simulink model "gm_parallel_lht"  (R2019b)
settings: Solver=FixedStepDiscrete  StartTime=0.0  StopTime=inf  RelTol=1e-3
undefined symbols (not defined in the file or in its folder): bt, height, width
libraries: hdlsllib x190, simulink x13, hdlmdlgenlib x7, dspsrcs4 x1
(part 8 of 18)

== system gm_parallel_lht/Parallel LHT/Parallel LHT Accumulator/Accumulator with Switches/Accumulator_instance72 ==
  mode : Inport  OutDataTypeStr=boolean  PortDimensions=1  SampleTime=6.66666666666667e-09
  address : Inport  Port=2  OutDataTypeStr=fixdt(0, 11, 0)  PortDimensions=1  SampleTime=6.66666666666667e-09
  edge : Inport  Port=3  OutDataTypeStr=boolean  PortDimensions=1  SampleTime=6.66666666666667e-09
  AND : Logic  IconShape=distinctive  AllPortsSameDT=off  OutDataTypeStr=boolean
  Add : Sum  OutDataTypeStr=fixdt(0, ceil(log2(maxRho*2)), 0)
  Block RAM : Subsystem
  Delay{,1..3} (4 alike) : Delay  DelayLength=1
  Multiport Switch : MultiPortSwitch  DataPortOrder=Zero-based contiguous  Inputs=2  zeroidx=on
  Multiport Switch1 : MultiPortSwitch  DataPortOrder=Zero-based contiguous  Inputs=2  zeroidx=on
  Relational Operator : RelationalOperator  Operator===  OutDataTypeStr=boolean  RndMeth=Simplest
  Vote : Constant  OutDataTypeStr=fixdt(0,1,0)  SampleTime=-1
  Zero : Constant  OutDataTypeStr=fixdt(0,1,0)  SampleTime=-1
  hps : Outport
  wires:
  Add/1 -> Delay3/1, Multiport Switch/3
  Multiport Switch1/1 -> Add/2
  Delay3/1 -> Multiport Switch1/3
  Multiport Switch/1 -> Block RAM/1(wr_data)
  edge/1 -> Delay1/1
  address/1 -> Block RAM/4(rd_addr), Delay/1, Relational Operator/2
  mode/1 -> Multiport Switch/1
  AND/1 -> Delay2/1
  Block RAM/1(rd_data) -> Multiport Switch1/2, hps/1
  Delay/1 -> Block RAM/2(wr_addr), Relational Operator/1
  Delay1/1 -> Block RAM/3(wr_en), AND/1
  Delay2/1 -> Multiport Switch1/1
  Relational Operator/1 -> AND/2
  Vote/1 -> Add/1
  Zero/1 -> Multiport Switch/2

== system gm_parallel_lht/Parallel LHT/Parallel LHT Accumulator/Accumulator with Switches/Accumulator_instance73 ==
  mode : Inport  OutDataTypeStr=boolean  PortDimensions=1  SampleTime=6.66666666666667e-09
  address : Inport  Port=2  OutDataTypeStr=fixdt(0, 11, 0)  PortDimensions=1  SampleTime=6.66666666666667e-09
  edge : Inport  Port=3  OutDataTypeStr=boolean  PortDimensions=1  SampleTime=6.66666666666667e-09
  AND : Logic  IconShape=distinctive  AllPortsSameDT=off  OutDataTypeStr=boolean
  Add : Sum  OutDataTypeStr=fixdt(0, ceil(log2(maxRho*2)), 0)
  Block RAM : Subsystem
  Delay{,1..3} (4 alike) : Delay  DelayLength=1
  Multiport Switch : MultiPortSwitch  DataPortOrder=Zero-based contiguous  Inputs=2  zeroidx=on
  Multiport Switch1 : MultiPortSwitch  DataPortOrder=Zero-based contiguous  Inputs=2  zeroidx=on
  Relational Operator : RelationalOperator  Operator===  OutDataTypeStr=boolean  RndMeth=Simplest
  Vote : Constant  OutDataTypeStr=fixdt(0,1,0)  SampleTime=-1
  Zero : Constant  OutDataTypeStr=fixdt(0,1,0)  SampleTime=-1
  hps : Outport
  wires:
  Add/1 -> Delay3/1, Multiport Switch/3
  Multiport Switch1/1 -> Add/2
  Delay3/1 -> Multiport Switch1/3
  Multiport Switch/1 -> Block RAM/1(wr_data)
  edge/1 -> Delay1/1
  address/1 -> Block RAM/4(rd_addr), Delay/1, Relational Operator/2
  mode/1 -> Multiport Switch/1
  AND/1 -> Delay2/1
  Block RAM/1(rd_data) -> Multiport Switch1/2, hps/1
  Delay/1 -> Block RAM/2(wr_addr), Relational Operator/1
  Delay1/1 -> Block RAM/3(wr_en), AND/1
  Delay2/1 -> Multiport Switch1/1
  Relational Operator/1 -> AND/2
  Vote/1 -> Add/1
  Zero/1 -> Multiport Switch/2

== system gm_parallel_lht/Parallel LHT/Parallel LHT Accumulator/Accumulator with Switches/Accumulator_instance74 ==
  mode : Inport  OutDataTypeStr=boolean  PortDimensions=1  SampleTime=6.66666666666667e-09
  address : Inport  Port=2  OutDataTypeStr=fixdt(0, 11, 0)  PortDimensions=1  SampleTime=6.66666666666667e-09
  edge : Inport  Port=3  OutDataTypeStr=boolean  PortDimensions=1  SampleTime=6.66666666666667e-09
  AND : Logic  IconShape=distinctive  AllPortsSameDT=off  OutDataTypeStr=boolean
  Add : Sum  OutDataTypeStr=fixdt(0, ceil(log2(maxRho*2)), 0)
  Block RAM : Subsystem
  Delay{,1..3} (4 alike) : Delay  DelayLength=1
  Multiport Switch : MultiPortSwitch  DataPortOrder=Zero-based contiguous  Inputs=2  zeroidx=on
  Multiport Switch1 : MultiPortSwitch  DataPortOrder=Zero-based contiguous  Inputs=2  zeroidx=on
  Relational Operator : RelationalOperator  Operator===  OutDataTypeStr=boolean  RndMeth=Simplest
  Vote : Constant  OutDataTypeStr=fixdt(0,1,0)  SampleTime=-1
  Zero : Constant  OutDataTypeStr=fixdt(0,1,0)  SampleTime=-1
  hps : Outport
  wires:
  Add/1 -> Delay3/1, Multiport Switch/3
  Multiport Switch1/1 -> Add/2
  Delay3/1 -> Multiport Switch1/3
  Multiport Switch/1 -> Block RAM/1(wr_data)
  edge/1 -> Delay1/1
  address/1 -> Block RAM/4(rd_addr), Delay/1, Relational Operator/2
  mode/1 -> Multiport Switch/1
  AND/1 -> Delay2/1
  Block RAM/1(rd_data) -> Multiport Switch1/2, hps/1
  Delay/1 -> Block RAM/2(wr_addr), Relational Operator/1
  Delay1/1 -> Block RAM/3(wr_en), AND/1
  Delay2/1 -> Multiport Switch1/1
  Relational Operator/1 -> AND/2
  Vote/1 -> Add/1
  Zero/1 -> Multiport Switch/2

== system gm_parallel_lht/Parallel LHT/Parallel LHT Accumulator/Accumulator with Switches/Accumulator_instance75 ==
  mode : Inport  OutDataTypeStr=boolean  PortDimensions=1  SampleTime=6.66666666666667e-09
  address : Inport  Port=2  OutDataTypeStr=fixdt(0, 11, 0)  PortDimensions=1  SampleTime=6.66666666666667e-09
  edge : Inport  Port=3  OutDataTypeStr=boolean  PortDimensions=1  SampleTime=6.66666666666667e-09
  AND : Logic  IconShape=distinctive  AllPortsSameDT=off  OutDataTypeStr=boolean
  Add : Sum  OutDataTypeStr=fixdt(0, ceil(log2(maxRho*2)), 0)
  Block RAM : Subsystem
  Delay{,1..3} (4 alike) : Delay  DelayLength=1
  Multiport Switch : MultiPortSwitch  DataPortOrder=Zero-based contiguous  Inputs=2  zeroidx=on
  Multiport Switch1 : MultiPortSwitch  DataPortOrder=Zero-based contiguous  Inputs=2  zeroidx=on
  Relational Operator : RelationalOperator  Operator===  OutDataTypeStr=boolean  RndMeth=Simplest
  Vote : Constant  OutDataTypeStr=fixdt(0,1,0)  SampleTime=-1
  Zero : Constant  OutDataTypeStr=fixdt(0,1,0)  SampleTime=-1
  hps : Outport
  wires:
  Add/1 -> Delay3/1, Multiport Switch/3
  Multiport Switch1/1 -> Add/2
  Delay3/1 -> Multiport Switch1/3
  Multiport Switch/1 -> Block RAM/1(wr_data)
  edge/1 -> Delay1/1
  address/1 -> Block RAM/4(rd_addr), Delay/1, Relational Operator/2
  mode/1 -> Multiport Switch/1
  AND/1 -> Delay2/1
  Block RAM/1(rd_data) -> Multiport Switch1/2, hps/1
  Delay/1 -> Block RAM/2(wr_addr), Relational Operator/1
  Delay1/1 -> Block RAM/3(wr_en), AND/1
  Delay2/1 -> Multiport Switch1/1
  Relational Operator/1 -> AND/2
  Vote/1 -> Add/1
  Zero/1 -> Multiport Switch/2

== system gm_parallel_lht/Parallel LHT/Parallel LHT Accumulator/Accumulator with Switches/Accumulator_instance76 ==
  mode : Inport  OutDataTypeStr=boolean  PortDimensions=1  SampleTime=6.66666666666667e-09
  address : Inport  Port=2  OutDataTypeStr=fixdt(0, 11, 0)  PortDimensions=1  SampleTime=6.66666666666667e-09
  edge : Inport  Port=3  OutDataTypeStr=boolean  PortDimensions=1  SampleTime=6.66666666666667e-09
  AND : Logic  IconShape=distinctive  AllPortsSameDT=off  OutDataTypeStr=boolean
  Add : Sum  OutDataTypeStr=fixdt(0, ceil(log2(maxRho*2)), 0)
  Block RAM : Subsystem
  Delay{,1..3} (4 alike) : Delay  DelayLength=1
  Multiport Switch : MultiPortSwitch  DataPortOrder=Zero-based contiguous  Inputs=2  zeroidx=on
  Multiport Switch1 : MultiPortSwitch  DataPortOrder=Zero-based contiguous  Inputs=2  zeroidx=on
  Relational Operator : RelationalOperator  Operator===  OutDataTypeStr=boolean  RndMeth=Simplest
  Vote : Constant  OutDataTypeStr=fixdt(0,1,0)  SampleTime=-1
  Zero : Constant  OutDataTypeStr=fixdt(0,1,0)  SampleTime=-1
  hps : Outport
  wires:
  Add/1 -> Delay3/1, Multiport Switch/3
  Multiport Switch1/1 -> Add/2
  Delay3/1 -> Multiport Switch1/3
  Multiport Switch/1 -> Block RAM/1(wr_data)
  edge/1 -> Delay1/1
  address/1 -> Block RAM/4(rd_addr), Delay/1, Relational Operator/2
  mode/1 -> Multiport Switch/1
  AND/1 -> Delay2/1
  Block RAM/1(rd_data) -> Multiport Switch1/2, hps/1
  Delay/1 -> Block RAM/2(wr_addr), Relational Operator/1
  Delay1/1 -> Block RAM/3(wr_en), AND/1
  Delay2/1 -> Multiport Switch1/1
  Relational Operator/1 -> AND/2
  Vote/1 -> Add/1
  Zero/1 -> Multiport Switch/2

== system gm_parallel_lht/Parallel LHT/Parallel LHT Accumulator/Accumulator with Switches/Accumulator_instance77 ==
  mode : Inport  OutDataTypeStr=boolean  PortDimensions=1  SampleTime=6.66666666666667e-09
  address : Inport  Port=2  OutDataTypeStr=fixdt(0, 11, 0)  PortDimensions=1  SampleTime=6.66666666666667e-09
  edge : Inport  Port=3  OutDataTypeStr=boolean  PortDimensions=1  SampleTime=6.66666666666667e-09
  AND : Logic  IconShape=distinctive  AllPortsSameDT=off  OutDataTypeStr=boolean
  Add : Sum  OutDataTypeStr=fixdt(0, ceil(log2(maxRho*2)), 0)
  Block RAM : Subsystem
  Delay{,1..3} (4 alike) : Delay  DelayLength=1
  Multiport Switch : MultiPortSwitch  DataPortOrder=Zero-based contiguous  Inputs=2  zeroidx=on
  Multiport Switch1 : MultiPortSwitch  DataPortOrder=Zero-based contiguous  Inputs=2  zeroidx=on
  Relational Operator : RelationalOperator  Operator===  OutDataTypeStr=boolean  RndMeth=Simplest
  Vote : Constant  OutDataTypeStr=fixdt(0,1,0)  SampleTime=-1
  Zero : Constant  OutDataTypeStr=fixdt(0,1,0)  SampleTime=-1
  hps : Outport
  wires:
  Add/1 -> Delay3/1, Multiport Switch/3
  Multiport Switch1/1 -> Add/2
  Delay3/1 -> Multiport Switch1/3
  Multiport Switch/1 -> Block RAM/1(wr_data)
  edge/1 -> Delay1/1
  address/1 -> Block RAM/4(rd_addr), Delay/1, Relational Operator/2
  mode/1 -> Multiport Switch/1
  AND/1 -> Delay2/1
  Block RAM/1(rd_data) -> Multiport Switch1/2, hps/1
  Delay/1 -> Block RAM/2(wr_addr), Relational Operator/1
  Delay1/1 -> Block RAM/3(wr_en), AND/1
  Delay2/1 -> Multiport Switch1/1
  Relational Operator/1 -> AND/2
  Vote/1 -> Add/1
  Zero/1 -> Multiport Switch/2

== system gm_parallel_lht/Parallel LHT/Parallel LHT Accumulator/Accumulator with Switches/Accumulator_instance78 ==
  mode : Inport  OutDataTypeStr=boolean  PortDimensions=1  SampleTime=6.66666666666667e-09
  address : Inport  Port=2  OutDataTypeStr=fixdt(0, 11, 0)  PortDimensions=1  SampleTime=6.66666666666667e-09
  edge : Inport  Port=3  OutDataTypeStr=boolean  PortDimensions=1  SampleTime=6.66666666666667e-09
  AND : Logic  IconShape=distinctive  AllPortsSameDT=off  OutDataTypeStr=boolean
  Add : Sum  OutDataTypeStr=fixdt(0, ceil(log2(maxRho*2)), 0)
  Block RAM : Subsystem
  Delay{,1..3} (4 alike) : Delay  DelayLength=1
  Multiport Switch : MultiPortSwitch  DataPortOrder=Zero-based contiguous  Inputs=2  zeroidx=on
  Multiport Switch1 : MultiPortSwitch  DataPortOrder=Zero-based contiguous  Inputs=2  zeroidx=on
  Relational Operator : RelationalOperator  Operator===  OutDataTypeStr=boolean  RndMeth=Simplest
  Vote : Constant  OutDataTypeStr=fixdt(0,1,0)  SampleTime=-1
  Zero : Constant  OutDataTypeStr=fixdt(0,1,0)  SampleTime=-1
  hps : Outport
  wires:
  Add/1 -> Delay3/1, Multiport Switch/3
  Multiport Switch1/1 -> Add/2
  Delay3/1 -> Multiport Switch1/3
  Multiport Switch/1 -> Block RAM/1(wr_data)
  edge/1 -> Delay1/1
  address/1 -> Block RAM/4(rd_addr), Delay/1, Relational Operator/2
  mode/1 -> Multiport Switch/1
  AND/1 -> Delay2/1
  Block RAM/1(rd_data) -> Multiport Switch1/2, hps/1
  Delay/1 -> Block RAM/2(wr_addr), Relational Operator/1
  Delay1/1 -> Block RAM/3(wr_en), AND/1
  Delay2/1 -> Multiport Switch1/1
  Relational Operator/1 -> AND/2
  Vote/1 -> Add/1
  Zero/1 -> Multiport Switch/2

== system gm_parallel_lht/Parallel LHT/Parallel LHT Accumulator/Accumulator with Switches/Accumulator_instance79 ==
  mode : Inport  OutDataTypeStr=boolean  PortDimensions=1  SampleTime=6.66666666666667e-09
  address : Inport  Port=2  OutDataTypeStr=fixdt(0, 11, 0)  PortDimensions=1  SampleTime=6.66666666666667e-09
  edge : Inport  Port=3  OutDataTypeStr=boolean  PortDimensions=1  SampleTime=6.66666666666667e-09
  AND : Logic  IconShape=distinctive  AllPortsSameDT=off  OutDataTypeStr=boolean
  Add : Sum  OutDataTypeStr=fixdt(0, ceil(log2(maxRho*2)), 0)
  Block RAM : Subsystem
  Delay{,1..3} (4 alike) : Delay  DelayLength=1
  Multiport Switch : MultiPortSwitch  DataPortOrder=Zero-based contiguous  Inputs=2  zeroidx=on
  Multiport Switch1 : MultiPortSwitch  DataPortOrder=Zero-based contiguous  Inputs=2  zeroidx=on
  Relational Operator : RelationalOperator  Operator===  OutDataTypeStr=boolean  RndMeth=Simplest
  Vote : Constant  OutDataTypeStr=fixdt(0,1,0)  SampleTime=-1
  Zero : Constant  OutDataTypeStr=fixdt(0,1,0)  SampleTime=-1
  hps : Outport
  wires:
  Add/1 -> Delay3/1, Multiport Switch/3
  Multiport Switch1/1 -> Add/2
  Delay3/1 -> Multiport Switch1/3
  Multiport Switch/1 -> Block RAM/1(wr_data)
  edge/1 -> Delay1/1
  address/1 -> Block RAM/4(rd_addr), Delay/1, Relational Operator/2
  mode/1 -> Multiport Switch/1
  AND/1 -> Delay2/1
  Block RAM/1(rd_data) -> Multiport Switch1/2, hps/1
  Delay/1 -> Block RAM/2(wr_addr), Relational Operator/1
  Delay1/1 -> Block RAM/3(wr_en), AND/1
  Delay2/1 -> Multiport Switch1/1
  Relational Operator/1 -> AND/2
  Vote/1 -> Add/1
  Zero/1 -> Multiport Switch/2

== system gm_parallel_lht/Parallel LHT/Parallel LHT Accumulator/Accumulator with Switches/Accumulator_instance8 ==
  mode : Inport  OutDataTypeStr=boolean  PortDimensions=1  SampleTime=6.66666666666667e-09
  address : Inport  Port=2  OutDataTypeStr=fixdt(0, 11, 0)  PortDimensions=1  SampleTime=6.66666666666667e-09
  edge : Inport  Port=3  OutDataTypeStr=boolean  PortDimensions=1  SampleTime=6.66666666666667e-09
  AND : Logic  IconShape=distinctive  AllPortsSameDT=off  OutDataTypeStr=boolean
  Add : Sum  OutDataTypeStr=fixdt(0, ceil(log2(maxRho*2)), 0)
  Block RAM : Subsystem
  Delay{,1..3} (4 alike) : Delay  DelayLength=1
  Multiport Switch : MultiPortSwitch  DataPortOrder=Zero-based contiguous  Inputs=2  zeroidx=on
  Multiport Switch1 : MultiPortSwitch  DataPortOrder=Zero-based contiguous  Inputs=2  zeroidx=on
  Relational Operator : RelationalOperator  Operator===  OutDataTypeStr=boolean  RndMeth=Simplest
  Vote : Constant  OutDataTypeStr=fixdt(0,1,0)  SampleTime=-1
  Zero : Constant  OutDataTypeStr=fixdt(0,1,0)  SampleTime=-1
  hps : Outport
  wires:
  Add/1 -> Delay3/1, Multiport Switch/3
  Multiport Switch1/1 -> Add/2
  Delay3/1 -> Multiport Switch1/3
  Multiport Switch/1 -> Block RAM/1(wr_data)
  edge/1 -> Delay1/1
  address/1 -> Block RAM/4(rd_addr), Delay/1, Relational Operator/2
  mode/1 -> Multiport Switch/1
  AND/1 -> Delay2/1
  Block RAM/1(rd_data) -> Multiport Switch1/2, hps/1
  Delay/1 -> Block RAM/2(wr_addr), Relational Operator/1
  Delay1/1 -> Block RAM/3(wr_en), AND/1
  Delay2/1 -> Multiport Switch1/1
  Relational Operator/1 -> AND/2
  Vote/1 -> Add/1
  Zero/1 -> Multiport Switch/2

== system gm_parallel_lht/Parallel LHT/Parallel LHT Accumulator/Accumulator with Switches/Accumulator_instance80 ==
  mode : Inport  OutDataTypeStr=boolean  PortDimensions=1  SampleTime=6.66666666666667e-09
  address : Inport  Port=2  OutDataTypeStr=fixdt(0, 11, 0)  PortDimensions=1  SampleTime=6.66666666666667e-09
  edge : Inport  Port=3  OutDataTypeStr=boolean  PortDimensions=1  SampleTime=6.66666666666667e-09
  AND : Logic  IconShape=distinctive  AllPortsSameDT=off  OutDataTypeStr=boolean
  Add : Sum  OutDataTypeStr=fixdt(0, ceil(log2(maxRho*2)), 0)
  Block RAM : Subsystem
  Delay{,1..3} (4 alike) : Delay  DelayLength=1
  Multiport Switch : MultiPortSwitch  DataPortOrder=Zero-based contiguous  Inputs=2  zeroidx=on
  Multiport Switch1 : MultiPortSwitch  DataPortOrder=Zero-based contiguous  Inputs=2  zeroidx=on
  Relational Operator : RelationalOperator  Operator===  OutDataTypeStr=boolean  RndMeth=Simplest
  Vote : Constant  OutDataTypeStr=fixdt(0,1,0)  SampleTime=-1
  Zero : Constant  OutDataTypeStr=fixdt(0,1,0)  SampleTime=-1
  hps : Outport
  wires:
  Add/1 -> Delay3/1, Multiport Switch/3
  Multiport Switch1/1 -> Add/2
  Delay3/1 -> Multiport Switch1/3
  Multiport Switch/1 -> Block RAM/1(wr_data)
  edge/1 -> Delay1/1
  address/1 -> Block RAM/4(rd_addr), Delay/1, Relational Operator/2
  mode/1 -> Multiport Switch/1
  AND/1 -> Delay2/1
  Block RAM/1(rd_data) -> Multiport Switch1/2, hps/1
  Delay/1 -> Block RAM/2(wr_addr), Relational Operator/1
  Delay1/1 -> Block RAM/3(wr_en), AND/1
  Delay2/1 -> Multiport Switch1/1
  Relational Operator/1 -> AND/2
  Vote/1 -> Add/1
  Zero/1 -> Multiport Switch/2

== system gm_parallel_lht/Parallel LHT/Parallel LHT Accumulator/Accumulator with Switches/Accumulator_instance81 ==
  mode : Inport  OutDataTypeStr=boolean  PortDimensions=1  SampleTime=6.66666666666667e-09
  address : Inport  Port=2  OutDataTypeStr=fixdt(0, 11, 0)  PortDimensions=1  SampleTime=6.66666666666667e-09
  edge : Inport  Port=3  OutDataTypeStr=boolean  PortDimensions=1  SampleTime=6.66666666666667e-09
  AND : Logic  IconShape=distinctive  AllPortsSameDT=off  OutDataTypeStr=boolean
  Add : Sum  OutDataTypeStr=fixdt(0, ceil(log2(maxRho*2)), 0)
  Block RAM : Subsystem
  Delay{,1..3} (4 alike) : Delay  DelayLength=1
  Multiport Switch : MultiPortSwitch  DataPortOrder=Zero-based contiguous  Inputs=2  zeroidx=on
  Multiport Switch1 : MultiPortSwitch  DataPortOrder=Zero-based contiguous  Inputs=2  zeroidx=on
  Relational Operator : RelationalOperator  Operator===  OutDataTypeStr=boolean  RndMeth=Simplest
  Vote : Constant  OutDataTypeStr=fixdt(0,1,0)  SampleTime=-1
  Zero : Constant  OutDataTypeStr=fixdt(0,1,0)  SampleTime=-1
  hps : Outport
  wires:
  Add/1 -> Delay3/1, Multiport Switch/3
  Multiport Switch1/1 -> Add/2
  Delay3/1 -> Multiport Switch1/3
  Multiport Switch/1 -> Block RAM/1(wr_data)
  edge/1 -> Delay1/1
  address/1 -> Block RAM/4(rd_addr), Delay/1, Relational Operator/2
  mode/1 -> Multiport Switch/1
  AND/1 -> Delay2/1
  Block RAM/1(rd_data) -> Multiport Switch1/2, hps/1
  Delay/1 -> Block RAM/2(wr_addr), Relational Operator/1
  Delay1/1 -> Block RAM/3(wr_en), AND/1
  Delay2/1 -> Multiport Switch1/1
  Relational Operator/1 -> AND/2
  Vote/1 -> Add/1
  Zero/1 -> Multiport Switch/2

== system gm_parallel_lht/Parallel LHT/Parallel LHT Accumulator/Accumulator with Switches/Accumulator_instance82 ==
  mode : Inport  OutDataTypeStr=boolean  PortDimensions=1  SampleTime=6.66666666666667e-09
  address : Inport  Port=2  OutDataTypeStr=fixdt(0, 11, 0)  PortDimensions=1  SampleTime=6.66666666666667e-09
  edge : Inport  Port=3  OutDataTypeStr=boolean  PortDimensions=1  SampleTime=6.66666666666667e-09
  AND : Logic  IconShape=distinctive  AllPortsSameDT=off  OutDataTypeStr=boolean
  Add : Sum  OutDataTypeStr=fixdt(0, ceil(log2(maxRho*2)), 0)
  Block RAM : Subsystem
  Delay{,1..3} (4 alike) : Delay  DelayLength=1
  Multiport Switch : MultiPortSwitch  DataPortOrder=Zero-based contiguous  Inputs=2  zeroidx=on
  Multiport Switch1 : MultiPortSwitch  DataPortOrder=Zero-based contiguous  Inputs=2  zeroidx=on
  Relational Operator : RelationalOperator  Operator===  OutDataTypeStr=boolean  RndMeth=Simplest
  Vote : Constant  OutDataTypeStr=fixdt(0,1,0)  SampleTime=-1
  Zero : Constant  OutDataTypeStr=fixdt(0,1,0)  SampleTime=-1
  hps : Outport
  wires:
  Add/1 -> Delay3/1, Multiport Switch/3
  Multiport Switch1/1 -> Add/2
  Delay3/1 -> Multiport Switch1/3
  Multiport Switch/1 -> Block RAM/1(wr_data)
  edge/1 -> Delay1/1
  address/1 -> Block RAM/4(rd_addr), Delay/1, Relational Operator/2
  mode/1 -> Multiport Switch/1
  AND/1 -> Delay2/1
  Block RAM/1(rd_data) -> Multiport Switch1/2, hps/1
  Delay/1 -> Block RAM/2(wr_addr), Relational Operator/1
  Delay1/1 -> Block RAM/3(wr_en), AND/1
  Delay2/1 -> Multiport Switch1/1
  Relational Operator/1 -> AND/2
  Vote/1 -> Add/1
  Zero/1 -> Multiport Switch/2

== system gm_parallel_lht/Parallel LHT/Parallel LHT Accumulator/Accumulator with Switches/Accumulator_instance83 ==
  mode : Inport  OutDataTypeStr=boolean  PortDimensions=1  SampleTime=6.66666666666667e-09
  address : Inport  Port=2  OutDataTypeStr=fixdt(0, 11, 0)  PortDimensions=1  SampleTime=6.66666666666667e-09
  edge : Inport  Port=3  OutDataTypeStr=boolean  PortDimensions=1  SampleTime=6.66666666666667e-09
  AND : Logic  IconShape=distinctive  AllPortsSameDT=off  OutDataTypeStr=boolean
  Add : Sum  OutDataTypeStr=fixdt(0, ceil(log2(maxRho*2)), 0)
  Block RAM : Subsystem
  Delay{,1..3} (4 alike) : Delay  DelayLength=1
  Multiport Switch : MultiPortSwitch  DataPortOrder=Zero-based contiguous  Inputs=2  zeroidx=on
  Multiport Switch1 : MultiPortSwitch  DataPortOrder=Zero-based contiguous  Inputs=2  zeroidx=on
  Relational Operator : RelationalOperator  Operator===  OutDataTypeStr=boolean  RndMeth=Simplest
  Vote : Constant  OutDataTypeStr=fixdt(0,1,0)  SampleTime=-1
  Zero : Constant  OutDataTypeStr=fixdt(0,1,0)  SampleTime=-1
  hps : Outport
  wires:
  Add/1 -> Delay3/1, Multiport Switch/3
  Multiport Switch1/1 -> Add/2
  Delay3/1 -> Multiport Switch1/3
  Multiport Switch/1 -> Block RAM/1(wr_data)
  edge/1 -> Delay1/1
  address/1 -> Block RAM/4(rd_addr), Delay/1, Relational Operator/2
  mode/1 -> Multiport Switch/1
  AND/1 -> Delay2/1
  Block RAM/1(rd_data) -> Multiport Switch1/2, hps/1
  Delay/1 -> Block RAM/2(wr_addr), Relational Operator/1
  Delay1/1 -> Block RAM/3(wr_en), AND/1
  Delay2/1 -> Multiport Switch1/1
  Relational Operator/1 -> AND/2
  Vote/1 -> Add/1
  Zero/1 -> Multiport Switch/2

== system gm_parallel_lht/Parallel LHT/Parallel LHT Accumulator/Accumulator with Switches/Accumulator_instance84 ==
  mode : Inport  OutDataTypeStr=boolean  PortDimensions=1  SampleTime=6.66666666666667e-09
  address : Inport  Port=2  OutDataTypeStr=fixdt(0, 11, 0)  PortDimensions=1  SampleTime=6.66666666666667e-09
  edge : Inport  Port=3  OutDataTypeStr=boolean  PortDimensions=1  SampleTime=6.66666666666667e-09
  AND : Logic  IconShape=distinctive  AllPortsSameDT=off  OutDataTypeStr=boolean
  Add : Sum  OutDataTypeStr=fixdt(0, ceil(log2(maxRho*2)), 0)
  Block RAM : Subsystem
  Delay{,1..3} (4 alike) : Delay  DelayLength=1
  Multiport Switch : MultiPortSwitch  DataPortOrder=Zero-based contiguous  Inputs=2  zeroidx=on
  Multiport Switch1 : MultiPortSwitch  DataPortOrder=Zero-based contiguous  Inputs=2  zeroidx=on
  Relational Operator : RelationalOperator  Operator===  OutDataTypeStr=boolean  RndMeth=Simplest
  Vote : Constant  OutDataTypeStr=fixdt(0,1,0)  SampleTime=-1
  Zero : Constant  OutDataTypeStr=fixdt(0,1,0)  SampleTime=-1
  hps : Outport
  wires:
  Add/1 -> Delay3/1, Multiport Switch/3
  Multiport Switch1/1 -> Add/2
  Delay3/1 -> Multiport Switch1/3
  Multiport Switch/1 -> Block RAM/1(wr_data)
  edge/1 -> Delay1/1
  address/1 -> Block RAM/4(rd_addr), Delay/1, Relational Operator/2
  mode/1 -> Multiport Switch/1
  AND/1 -> Delay2/1
  Block RAM/1(rd_data) -> Multiport Switch1/2, hps/1
  Delay/1 -> Block RAM/2(wr_addr), Relational Operator/1
  Delay1/1 -> Block RAM/3(wr_en), AND/1
  Delay2/1 -> Multiport Switch1/1
  Relational Operator/1 -> AND/2
  Vote/1 -> Add/1
  Zero/1 -> Multiport Switch/2

== system gm_parallel_lht/Parallel LHT/Parallel LHT Accumulator/Accumulator with Switches/Accumulator_instance85 ==
  mode : Inport  OutDataTypeStr=boolean  PortDimensions=1  SampleTime=6.66666666666667e-09
  address : Inport  Port=2  OutDataTypeStr=fixdt(0, 11, 0)  PortDimensions=1  SampleTime=6.66666666666667e-09
  edge : Inport  Port=3  OutDataTypeStr=boolean  PortDimensions=1  SampleTime=6.66666666666667e-09
  AND : Logic  IconShape=distinctive  AllPortsSameDT=off  OutDataTypeStr=boolean
  Add : Sum  OutDataTypeStr=fixdt(0, ceil(log2(maxRho*2)), 0)
  Block RAM : Subsystem
  Delay{,1..3} (4 alike) : Delay  DelayLength=1
  Multiport Switch : MultiPortSwitch  DataPortOrder=Zero-based contiguous  Inputs=2  zeroidx=on
  Multiport Switch1 : MultiPortSwitch  DataPortOrder=Zero-based contiguous  Inputs=2  zeroidx=on
  Relational Operator : RelationalOperator  Operator===  OutDataTypeStr=boolean  RndMeth=Simplest
  Vote : Constant  OutDataTypeStr=fixdt(0,1,0)  SampleTime=-1
  Zero : Constant  OutDataTypeStr=fixdt(0,1,0)  SampleTime=-1
  hps : Outport
  wires:
  Add/1 -> Delay3/1, Multiport Switch/3
  Multiport Switch1/1 -> Add/2
  Delay3/1 -> Multiport Switch1/3
  Multiport Switch/1 -> Block RAM/1(wr_data)
  edge/1 -> Delay1/1
  address/1 -> Block RAM/4(rd_addr), Delay/1, Relational Operator/2
  mode/1 -> Multiport Switch/1
  AND/1 -> Delay2/1
  Block RAM/1(rd_data) -> Multiport Switch1/2, hps/1
  Delay/1 -> Block RAM/2(wr_addr), Relational Operator/1
  Delay1/1 -> Block RAM/3(wr_en), AND/1
  Delay2/1 -> Multiport Switch1/1
  Relational Operator/1 -> AND/2
  Vote/1 -> Add/1
  Zero/1 -> Multiport Switch/2

== system gm_parallel_lht/Parallel LHT/Parallel LHT Accumulator/Accumulator with Switches/Accumulator_instance86 ==
  mode : Inport  OutDataTypeStr=boolean  PortDimensions=1  SampleTime=6.66666666666667e-09
  address : Inport  Port=2  OutDataTypeStr=fixdt(0, 11, 0)  PortDimensions=1  SampleTime=6.66666666666667e-09
  edge : Inport  Port=3  OutDataTypeStr=boolean  PortDimensions=1  SampleTime=6.66666666666667e-09
  AND : Logic  IconShape=distinctive  AllPortsSameDT=off  OutDataTypeStr=boolean
  Add : Sum  OutDataTypeStr=fixdt(0, ceil(log2(maxRho*2)), 0)
  Block RAM : Subsystem
  Delay{,1..3} (4 alike) : Delay  DelayLength=1
  Multiport Switch : MultiPortSwitch  DataPortOrder=Zero-based contiguous  Inputs=2  zeroidx=on
  Multiport Switch1 : MultiPortSwitch  DataPortOrder=Zero-based contiguous  Inputs=2  zeroidx=on
  Relational Operator : RelationalOperator  Operator===  OutDataTypeStr=boolean  RndMeth=Simplest
  Vote : Constant  OutDataTypeStr=fixdt(0,1,0)  SampleTime=-1
  Zero : Constant  OutDataTypeStr=fixdt(0,1,0)  SampleTime=-1
  hps : Outport
  wires:
  Add/1 -> Delay3/1, Multiport Switch/3
  Multiport Switch1/1 -> Add/2
  Delay3/1 -> Multiport Switch1/3
  Multiport Switch/1 -> Block RAM/1(wr_data)
  edge/1 -> Delay1/1
  address/1 -> Block RAM/4(rd_addr), Delay/1, Relational Operator/2
  mode/1 -> Multiport Switch/1
  AND/1 -> Delay2/1
  Block RAM/1(rd_data) -> Multiport Switch1/2, hps/1
  Delay/1 -> Block RAM/2(wr_addr), Relational Operator/1
  Delay1/1 -> Block RAM/3(wr_en), AND/1
  Delay2/1 -> Multiport Switch1/1
  Relational Operator/1 -> AND/2
  Vote/1 -> Add/1
  Zero/1 -> Multiport Switch/2

== system gm_parallel_lht/Parallel LHT/Parallel LHT Accumulator/Accumulator with Switches/Accumulator_instance87 ==
  mode : Inport  OutDataTypeStr=boolean  PortDimensions=1  SampleTime=6.66666666666667e-09
  address : Inport  Port=2  OutDataTypeStr=fixdt(0, 11, 0)  PortDimensions=1  SampleTime=6.66666666666667e-09
  edge : Inport  Port=3  OutDataTypeStr=boolean  PortDimensions=1  SampleTime=6.66666666666667e-09
  AND : Logic  IconShape=distinctive  AllPortsSameDT=off  OutDataTypeStr=boolean
  Add : Sum  OutDataTypeStr=fixdt(0, ceil(log2(maxRho*2)), 0)
  Block RAM : Subsystem
  Delay{,1..3} (4 alike) : Delay  DelayLength=1
  Multiport Switch : MultiPortSwitch  DataPortOrder=Zero-based contiguous  Inputs=2  zeroidx=on
  Multiport Switch1 : MultiPortSwitch  DataPortOrder=Zero-based contiguous  Inputs=2  zeroidx=on
  Relational Operator : RelationalOperator  Operator===  OutDataTypeStr=boolean  RndMeth=Simplest
  Vote : Constant  OutDataTypeStr=fixdt(0,1,0)  SampleTime=-1
  Zero : Constant  OutDataTypeStr=fixdt(0,1,0)  SampleTime=-1
  hps : Outport
  wires:
  Add/1 -> Delay3/1, Multiport Switch/3
  Multiport Switch1/1 -> Add/2
  Delay3/1 -> Multiport Switch1/3
  Multiport Switch/1 -> Block RAM/1(wr_data)
  edge/1 -> Delay1/1
  address/1 -> Block RAM/4(rd_addr), Delay/1, Relational Operator/2
  mode/1 -> Multiport Switch/1
  AND/1 -> Delay2/1
  Block RAM/1(rd_data) -> Multiport Switch1/2, hps/1
  Delay/1 -> Block RAM/2(wr_addr), Relational Operator/1
  Delay1/1 -> Block RAM/3(wr_en), AND/1
  Delay2/1 -> Multiport Switch1/1
  Relational Operator/1 -> AND/2
  Vote/1 -> Add/1
  Zero/1 -> Multiport Switch/2

== system gm_parallel_lht/Parallel LHT/Parallel LHT Accumulator/Accumulator with Switches/Accumulator_instance88 ==
  mode : Inport  OutDataTypeStr=boolean  PortDimensions=1  SampleTime=6.66666666666667e-09
  address : Inport  Port=2  OutDataTypeStr=fixdt(0, 11, 0)  PortDimensions=1  SampleTime=6.66666666666667e-09
  edge : Inport  Port=3  OutDataTypeStr=boolean  PortDimensions=1  SampleTime=6.66666666666667e-09
  AND : Logic  IconShape=distinctive  AllPortsSameDT=off  OutDataTypeStr=boolean
  Add : Sum  OutDataTypeStr=fixdt(0, ceil(log2(maxRho*2)), 0)
  Block RAM : Subsystem
  Delay{,1..3} (4 alike) : Delay  DelayLength=1
  Multiport Switch : MultiPortSwitch  DataPortOrder=Zero-based contiguous  Inputs=2  zeroidx=on
  Multiport Switch1 : MultiPortSwitch  DataPortOrder=Zero-based contiguous  Inputs=2  zeroidx=on
  Relational Operator : RelationalOperator  Operator===  OutDataTypeStr=boolean  RndMeth=Simplest
  Vote : Constant  OutDataTypeStr=fixdt(0,1,0)  SampleTime=-1
  Zero : Constant  OutDataTypeStr=fixdt(0,1,0)  SampleTime=-1
  hps : Outport
  wires:
  Add/1 -> Delay3/1, Multiport Switch/3
  Multiport Switch1/1 -> Add/2
  Delay3/1 -> Multiport Switch1/3
  Multiport Switch/1 -> Block RAM/1(wr_data)
  edge/1 -> Delay1/1
  address/1 -> Block RAM/4(rd_addr), Delay/1, Relational Operator/2
  mode/1 -> Multiport Switch/1
  AND/1 -> Delay2/1
  Block RAM/1(rd_data) -> Multiport Switch1/2, hps/1
  Delay/1 -> Block RAM/2(wr_addr), Relational Operator/1
  Delay1/1 -> Block RAM/3(wr_en), AND/1
  Delay2/1 -> Multiport Switch1/1
  Relational Operator/1 -> AND/2
  Vote/1 -> Add/1
  Zero/1 -> Multiport Switch/2

== system gm_parallel_lht/Parallel LHT/Parallel LHT Accumulator/Accumulator with Switches/Accumulator_instance89 ==
  mode : Inport  OutDataTypeStr=boolean  PortDimensions=1  SampleTime=6.66666666666667e-09
  address : Inport  Port=2  OutDataTypeStr=fixdt(0, 11, 0)  PortDimensions=1  SampleTime=6.66666666666667e-09
  edge : Inport  Port=3  OutDataTypeStr=boolean  PortDimensions=1  SampleTime=6.66666666666667e-09
  AND : Logic  IconShape=distinctive  AllPortsSameDT=off  OutDataTypeStr=boolean
  Add : Sum  OutDataTypeStr=fixdt(0, ceil(log2(maxRho*2)), 0)
  Block RAM : Subsystem
  Delay{,1..3} (4 alike) : Delay  DelayLength=1
  Multiport Switch : MultiPortSwitch  DataPortOrder=Zero-based contiguous  Inputs=2  zeroidx=on
  Multiport Switch1 : MultiPortSwitch  DataPortOrder=Zero-based contiguous  Inputs=2  zeroidx=on
  Relational Operator : RelationalOperator  Operator===  OutDataTypeStr=boolean  RndMeth=Simplest
  Vote : Constant  OutDataTypeStr=fixdt(0,1,0)  SampleTime=-1
  Zero : Constant  OutDataTypeStr=fixdt(0,1,0)  SampleTime=-1
  hps : Outport
  wires:
  Add/1 -> Delay3/1, Multiport Switch/3
  Multiport Switch1/1 -> Add/2
  Delay3/1 -> Multiport Switch1/3
  Multiport Switch/1 -> Block RAM/1(wr_data)
  edge/1 -> Delay1/1
  address/1 -> Block RAM/4(rd_addr), Delay/1, Relational Operator/2
  mode/1 -> Multiport Switch/1
  AND/1 -> Delay2/1
  Block RAM/1(rd_data) -> Multiport Switch1/2, hps/1
  Delay/1 -> Block RAM/2(wr_addr), Relational Operator/1
  Delay1/1 -> Block RAM/3(wr_en), AND/1
  Delay2/1 -> Multiport Switch1/1
  Relational Operator/1 -> AND/2
  Vote/1 -> Add/1
  Zero/1 -> Multiport Switch/2

== system gm_parallel_lht/Parallel LHT/Parallel LHT Accumulator/Accumulator with Switches/Accumulator_instance9 ==
  mode : Inport  OutDataTypeStr=boolean  PortDimensions=1  SampleTime=6.66666666666667e-09
  address : Inport  Port=2  OutDataTypeStr=fixdt(0, 11, 0)  PortDimensions=1  SampleTime=6.66666666666667e-09
  edge : Inport  Port=3  OutDataTypeStr=boolean  PortDimensions=1  SampleTime=6.66666666666667e-09
  AND : Logic  IconShape=distinctive  AllPortsSameDT=off  OutDataTypeStr=boolean
  Add : Sum  OutDataTypeStr=fixdt(0, ceil(log2(maxRho*2)), 0)
  Block RAM : Subsystem
  Delay{,1..3} (4 alike) : Delay  DelayLength=1
  Multiport Switch : MultiPortSwitch  DataPortOrder=Zero-based contiguous  Inputs=2  zeroidx=on
  Multiport Switch1 : MultiPortSwitch  DataPortOrder=Zero-based contiguous  Inputs=2  zeroidx=on
  Relational Operator : RelationalOperator  Operator===  OutDataTypeStr=boolean  RndMeth=Simplest
  Vote : Constant  OutDataTypeStr=fixdt(0,1,0)  SampleTime=-1
  Zero : Constant  OutDataTypeStr=fixdt(0,1,0)  SampleTime=-1
  hps : Outport
  wires:
  Add/1 -> Delay3/1, Multiport Switch/3
  Multiport Switch1/1 -> Add/2
  Delay3/1 -> Multiport Switch1/3
  Multiport Switch/1 -> Block RAM/1(wr_data)
  edge/1 -> Delay1/1
  address/1 -> Block RAM/4(rd_addr), Delay/1, Relational Operator/2
  mode/1 -> Multiport Switch/1
  AND/1 -> Delay2/1
  Block RAM/1(rd_data) -> Multiport Switch1/2, hps/1
  Delay/1 -> Block RAM/2(wr_addr), Relational Operator/1
  Delay1/1 -> Block RAM/3(wr_en), AND/1
  Delay2/1 -> Multiport Switch1/1
  Relational Operator/1 -> AND/2
  Vote/1 -> Add/1
  Zero/1 -> Multiport Switch/2

== system gm_parallel_lht/Parallel LHT/Parallel LHT Accumulator/Accumulator with Switches/Accumulator_instance90 ==
  mode : Inport  OutDataTypeStr=boolean  PortDimensions=1  SampleTime=6.66666666666667e-09
  address : Inport  Port=2  OutDataTypeStr=fixdt(0, 11, 0)  PortDimensions=1  SampleTime=6.66666666666667e-09
  edge : Inport  Port=3  OutDataTypeStr=boolean  PortDimensions=1  SampleTime=6.66666666666667e-09
  AND : Logic  IconShape=distinctive  AllPortsSameDT=off  OutDataTypeStr=boolean
  Add : Sum  OutDataTypeStr=fixdt(0, ceil(log2(maxRho*2)), 0)
  Block RAM : Subsystem
  Delay{,1..3} (4 alike) : Delay  DelayLength=1
  Multiport Switch : MultiPortSwitch  DataPortOrder=Zero-based contiguous  Inputs=2  zeroidx=on
  Multiport Switch1 : MultiPortSwitch  DataPortOrder=Zero-based contiguous  Inputs=2  zeroidx=on
  Relational Operator : RelationalOperator  Operator===  OutDataTypeStr=boolean  RndMeth=Simplest
  Vote : Constant  OutDataTypeStr=fixdt(0,1,0)  SampleTime=-1
  Zero : Constant  OutDataTypeStr=fixdt(0,1,0)  SampleTime=-1
  hps : Outport
  wires:
  Add/1 -> Delay3/1, Multiport Switch/3
  Multiport Switch1/1 -> Add/2
  Delay3/1 -> Multiport Switch1/3
  Multiport Switch/1 -> Block RAM/1(wr_data)
  edge/1 -> Delay1/1
  address/1 -> Block RAM/4(rd_addr), Delay/1, Relational Operator/2
  mode/1 -> Multiport Switch/1
  AND/1 -> Delay2/1
  Block RAM/1(rd_data) -> Multiport Switch1/2, hps/1
  Delay/1 -> Block RAM/2(wr_addr), Relational Operator/1
  Delay1/1 -> Block RAM/3(wr_en), AND/1
  Delay2/1 -> Multiport Switch1/1
  Relational Operator/1 -> AND/2
  Vote/1 -> Add/1
  Zero/1 -> Multiport Switch/2

== system gm_parallel_lht/Parallel LHT/Parallel LHT Accumulator/Accumulator with Switches/Accumulator_instance91 ==
  mode : Inport  OutDataTypeStr=boolean  PortDimensions=1  SampleTime=6.66666666666667e-09
  address : Inport  Port=2  OutDataTypeStr=fixdt(0, 11, 0)  PortDimensions=1  SampleTime=6.66666666666667e-09
  edge : Inport  Port=3  OutDataTypeStr=boolean  PortDimensions=1  SampleTime=6.66666666666667e-09
  AND : Logic  IconShape=distinctive  AllPortsSameDT=off  OutDataTypeStr=boolean
  Add : Sum  OutDataTypeStr=fixdt(0, ceil(log2(maxRho*2)), 0)
  Block RAM : Subsystem
  Delay{,1..3} (4 alike) : Delay  DelayLength=1
  Multiport Switch : MultiPortSwitch  DataPortOrder=Zero-based contiguous  Inputs=2  zeroidx=on
  Multiport Switch1 : MultiPortSwitch  DataPortOrder=Zero-based contiguous  Inputs=2  zeroidx=on
  Relational Operator : RelationalOperator  Operator===  OutDataTypeStr=boolean  RndMeth=Simplest
  Vote : Constant  OutDataTypeStr=fixdt(0,1,0)  SampleTime=-1
  Zero : Constant  OutDataTypeStr=fixdt(0,1,0)  SampleTime=-1
  hps : Outport
  wires:
  Add/1 -> Delay3/1, Multiport Switch/3
  Multiport Switch1/1 -> Add/2
  Delay3/1 -> Multiport Switch1/3
  Multiport Switch/1 -> Block RAM/1(wr_data)
  edge/1 -> Delay1/1
  address/1 -> Block RAM/4(rd_addr), Delay/1, Relational Operator/2
  mode/1 -> Multiport Switch/1
  AND/1 -> Delay2/1
  Block RAM/1(rd_data) -> Multiport Switch1/2, hps/1
  Delay/1 -> Block RAM/2(wr_addr), Relational Operator/1
  Delay1/1 -> Block RAM/3(wr_en), AND/1
  Delay2/1 -> Multiport Switch1/1
  Relational Operator/1 -> AND/2
  Vote/1 -> Add/1
  Zero/1 -> Multiport Switch/2

== system gm_parallel_lht/Parallel LHT/Parallel LHT Accumulator/Accumulator with Switches/Accumulator_instance92 ==
  mode : Inport  OutDataTypeStr=boolean  PortDimensions=1  SampleTime=6.66666666666667e-09
  address : Inport  Port=2  OutDataTypeStr=fixdt(0, 11, 0)  PortDimensions=1  SampleTime=6.66666666666667e-09
  edge : Inport  Port=3  OutDataTypeStr=boolean  PortDimensions=1  SampleTime=6.66666666666667e-09
  AND : Logic  IconShape=distinctive  AllPortsSameDT=off  OutDataTypeStr=boolean
  Add : Sum  OutDataTypeStr=fixdt(0, ceil(log2(maxRho*2)), 0)
  Block RAM : Subsystem
  Delay{,1..3} (4 alike) : Delay  DelayLength=1
  Multiport Switch : MultiPortSwitch  DataPortOrder=Zero-based contiguous  Inputs=2  zeroidx=on
  Multiport Switch1 : MultiPortSwitch  DataPortOrder=Zero-based contiguous  Inputs=2  zeroidx=on
  Relational Operator : RelationalOperator  Operator===  OutDataTypeStr=boolean  RndMeth=Simplest
  Vote : Constant  OutDataTypeStr=fixdt(0,1,0)  SampleTime=-1
  Zero : Constant  OutDataTypeStr=fixdt(0,1,0)  SampleTime=-1
  hps : Outport
  wires:
  Add/1 -> Delay3/1, Multiport Switch/3
  Multiport Switch1/1 -> Add/2
  Delay3/1 -> Multiport Switch1/3
  Multiport Switch/1 -> Block RAM/1(wr_data)
  edge/1 -> Delay1/1
  address/1 -> Block RAM/4(rd_addr), Delay/1, Relational Operator/2
  mode/1 -> Multiport Switch/1
  AND/1 -> Delay2/1
  Block RAM/1(rd_data) -> Multiport Switch1/2, hps/1
  Delay/1 -> Block RAM/2(wr_addr), Relational Operator/1
  Delay1/1 -> Block RAM/3(wr_en), AND/1
  Delay2/1 -> Multiport Switch1/1
  Relational Operator/1 -> AND/2
  Vote/1 -> Add/1
  Zero/1 -> Multiport Switch/2

== system gm_parallel_lht/Parallel LHT/Parallel LHT Accumulator/Accumulator with Switches/Accumulator_instance93 ==
  mode : Inport  OutDataTypeStr=boolean  PortDimensions=1  SampleTime=6.66666666666667e-09
  address : Inport  Port=2  OutDataTypeStr=fixdt(0, 11, 0)  PortDimensions=1  SampleTime=6.66666666666667e-09
  edge : Inport  Port=3  OutDataTypeStr=boolean  PortDimensions=1  SampleTime=6.66666666666667e-09
  AND : Logic  IconShape=distinctive  AllPortsSameDT=off  OutDataTypeStr=boolean
  Add : Sum  OutDataTypeStr=fixdt(0, ceil(log2(maxRho*2)), 0)
  Block RAM : Subsystem
  Delay{,1..3} (4 alike) : Delay  DelayLength=1
  Multiport Switch : MultiPortSwitch  DataPortOrder=Zero-based contiguous  Inputs=2  zeroidx=on
  Multiport Switch1 : MultiPortSwitch  DataPortOrder=Zero-based contiguous  Inputs=2  zeroidx=on
  Relational Operator : RelationalOperator  Operator===  OutDataTypeStr=boolean  RndMeth=Simplest
  Vote : Constant  OutDataTypeStr=fixdt(0,1,0)  SampleTime=-1
  Zero : Constant  OutDataTypeStr=fixdt(0,1,0)  SampleTime=-1
  hps : Outport
  wires:
  Add/1 -> Delay3/1, Multiport Switch/3
  Multiport Switch1/1 -> Add/2
  Delay3/1 -> Multiport Switch1/3
  Multiport Switch/1 -> Block RAM/1(wr_data)
  edge/1 -> Delay1/1
  address/1 -> Block RAM/4(rd_addr), Delay/1, Relational Operator/2
  mode/1 -> Multiport Switch/1
  AND/1 -> Delay2/1
  Block RAM/1(rd_data) -> Multiport Switch1/2, hps/1
  Delay/1 -> Block RAM/2(wr_addr), Relational Operator/1
  Delay1/1 -> Block RAM/3(wr_en), AND/1
  Delay2/1 -> Multiport Switch1/1
  Relational Operator/1 -> AND/2
  Vote/1 -> Add/1
  Zero/1 -> Multiport Switch/2

== system gm_parallel_lht/Parallel LHT/Parallel LHT Accumulator/Accumulator with Switches/Accumulator_instance94 ==
  mode : Inport  OutDataTypeStr=boolean  PortDimensions=1  SampleTime=6.66666666666667e-09
  address : Inport  Port=2  OutDataTypeStr=fixdt(0, 11, 0)  PortDimensions=1  SampleTime=6.66666666666667e-09
  edge : Inport  Port=3  OutDataTypeStr=boolean  PortDimensions=1  SampleTime=6.66666666666667e-09
  AND : Logic  IconShape=distinctive  AllPortsSameDT=off  OutDataTypeStr=boolean
  Add : Sum  OutDataTypeStr=fixdt(0, ceil(log2(maxRho*2)), 0)
  Block RAM : Subsystem
  Delay{,1..3} (4 alike) : Delay  DelayLength=1
  Multiport Switch : MultiPortSwitch  DataPortOrder=Zero-based contiguous  Inputs=2  zeroidx=on
  Multiport Switch1 : MultiPortSwitch  DataPortOrder=Zero-based contiguous  Inputs=2  zeroidx=on
  Relational Operator : RelationalOperator  Operator===  OutDataTypeStr=boolean  RndMeth=Simplest
  Vote : Constant  OutDataTypeStr=fixdt(0,1,0)  SampleTime=-1
  Zero : Constant  OutDataTypeStr=fixdt(0,1,0)  SampleTime=-1
  hps : Outport
  wires:
  Add/1 -> Delay3/1, Multiport Switch/3
  Multiport Switch1/1 -> Add/2
  Delay3/1 -> Multiport Switch1/3
  Multiport Switch/1 -> Block RAM/1(wr_data)
  edge/1 -> Delay1/1
  address/1 -> Block RAM/4(rd_addr), Delay/1, Relational Operator/2
  mode/1 -> Multiport Switch/1
  AND/1 -> Delay2/1
  Block RAM/1(rd_data) -> Multiport Switch1/2, hps/1
  Delay/1 -> Block RAM/2(wr_addr), Relational Operator/1
  Delay1/1 -> Block RAM/3(wr_en), AND/1
  Delay2/1 -> Multiport Switch1/1
  Relational Operator/1 -> AND/2
  Vote/1 -> Add/1
  Zero/1 -> Multiport Switch/2

== system gm_parallel_lht/Parallel LHT/Parallel LHT Accumulator/Accumulator with Switches/Accumulator_instance95 ==
  mode : Inport  OutDataTypeStr=boolean  PortDimensions=1  SampleTime=6.66666666666667e-09
  address : Inport  Port=2  OutDataTypeStr=fixdt(0, 11, 0)  PortDimensions=1  SampleTime=6.66666666666667e-09
  edge : Inport  Port=3  OutDataTypeStr=boolean  PortDimensions=1  SampleTime=6.66666666666667e-09
  AND : Logic  IconShape=distinctive  AllPortsSameDT=off  OutDataTypeStr=boolean
  Add : Sum  OutDataTypeStr=fixdt(0, ceil(log2(maxRho*2)), 0)
  Block RAM : Subsystem
  Delay{,1..3} (4 alike) : Delay  DelayLength=1
  Multiport Switch : MultiPortSwitch  DataPortOrder=Zero-based contiguous  Inputs=2  zeroidx=on
  Multiport Switch1 : MultiPortSwitch  DataPortOrder=Zero-based contiguous  Inputs=2  zeroidx=on
  Relational Operator : RelationalOperator  Operator===  OutDataTypeStr=boolean  RndMeth=Simplest
  Vote : Constant  OutDataTypeStr=fixdt(0,1,0)  SampleTime=-1
  Zero : Constant  OutDataTypeStr=fixdt(0,1,0)  SampleTime=-1
  hps : Outport
  wires:
  Add/1 -> Delay3/1, Multiport Switch/3
  Multiport Switch1/1 -> Add/2
  Delay3/1 -> Multiport Switch1/3
  Multiport Switch/1 -> Block RAM/1(wr_data)
  edge/1 -> Delay1/1
  address/1 -> Block RAM/4(rd_addr), Delay/1, Relational Operator/2
  mode/1 -> Multiport Switch/1
  AND/1 -> Delay2/1
  Block RAM/1(rd_data) -> Multiport Switch1/2, hps/1
  Delay/1 -> Block RAM/2(wr_addr), Relational Operator/1
  Delay1/1 -> Block RAM/3(wr_en), AND/1
  Delay2/1 -> Multiport Switch1/1
  Relational Operator/1 -> AND/2
  Vote/1 -> Add/1
  Zero/1 -> Multiport Switch/2

== system gm_parallel_lht/Parallel LHT/Parallel LHT Accumulator/Accumulator with Switches/Accumulator_instance96 ==
  mode : Inport  OutDataTypeStr=boolean  PortDimensions=1  SampleTime=6.66666666666667e-09
  address : Inport  Port=2  OutDataTypeStr=fixdt(0, 11, 0)  PortDimensions=1  SampleTime=6.66666666666667e-09
  edge : Inport  Port=3  OutDataTypeStr=boolean  PortDimensions=1  SampleTime=6.66666666666667e-09
  AND : Logic  IconShape=distinctive  AllPortsSameDT=off  OutDataTypeStr=boolean
  Add : Sum  OutDataTypeStr=fixdt(0, ceil(log2(maxRho*2)), 0)
  Block RAM : Subsystem
  Delay{,1..3} (4 alike) : Delay  DelayLength=1
  Multiport Switch : MultiPortSwitch  DataPortOrder=Zero-based contiguous  Inputs=2  zeroidx=on
  Multiport Switch1 : MultiPortSwitch  DataPortOrder=Zero-based contiguous  Inputs=2  zeroidx=on
  Relational Operator : RelationalOperator  Operator===  OutDataTypeStr=boolean  RndMeth=Simplest
  Vote : Constant  OutDataTypeStr=fixdt(0,1,0)  SampleTime=-1
  Zero : Constant  OutDataTypeStr=fixdt(0,1,0)  SampleTime=-1
  hps : Outport
  wires:
  Add/1 -> Delay3/1, Multiport Switch/3
  Multiport Switch1/1 -> Add/2
  Delay3/1 -> Multiport Switch1/3
  Multiport Switch/1 -> Block RAM/1(wr_data)
  edge/1 -> Delay1/1
  address/1 -> Block RAM/4(rd_addr), Delay/1, Relational Operator/2
  mode/1 -> Multiport Switch/1
  AND/1 -> Delay2/1
  Block RAM/1(rd_data) -> Multiport Switch1/2, hps/1
  Delay/1 -> Block RAM/2(wr_addr), Relational Operator/1
  Delay1/1 -> Block RAM/3(wr_en), AND/1
  Delay2/1 -> Multiport Switch1/1
  Relational Operator/1 -> AND/2
  Vote/1 -> Add/1
  Zero/1 -> Multiport Switch/2

== system gm_parallel_lht/Parallel LHT/Parallel LHT Accumulator/Accumulator with Switches/Accumulator_instance97 ==
  mode : Inport  OutDataTypeStr=boolean  PortDimensions=1  SampleTime=6.66666666666667e-09
  address : Inport  Port=2  OutDataTypeStr=fixdt(0, 11, 0)  PortDimensions=1  SampleTime=6.66666666666667e-09
  edge : Inport  Port=3  OutDataTypeStr=boolean  PortDimensions=1  SampleTime=6.66666666666667e-09
  AND : Logic  IconShape=distinctive  AllPortsSameDT=off  OutDataTypeStr=boolean
  Add : Sum  OutDataTypeStr=fixdt(0, ceil(log2(maxRho*2)), 0)
  Block RAM : Subsystem
  Delay{,1..3} (4 alike) : Delay  DelayLength=1
  Multiport Switch : MultiPortSwitch  DataPortOrder=Zero-based contiguous  Inputs=2  zeroidx=on
  Multiport Switch1 : MultiPortSwitch  DataPortOrder=Zero-based contiguous  Inputs=2  zeroidx=on
  Relational Operator : RelationalOperator  Operator===  OutDataTypeStr=boolean  RndMeth=Simplest
  Vote : Constant  OutDataTypeStr=fixdt(0,1,0)  SampleTime=-1
  Zero : Constant  OutDataTypeStr=fixdt(0,1,0)  SampleTime=-1
  hps : Outport
  wires:
  Add/1 -> Delay3/1, Multiport Switch/3
  Multiport Switch1/1 -> Add/2
  Delay3/1 -> Multiport Switch1/3
  Multiport Switch/1 -> Block RAM/1(wr_data)
  edge/1 -> Delay1/1
  address/1 -> Block RAM/4(rd_addr), Delay/1, Relational Operator/2
  mode/1 -> Multiport Switch/1
  AND/1 -> Delay2/1
  Block RAM/1(rd_data) -> Multiport Switch1/2, hps/1
  Delay/1 -> Block RAM/2(wr_addr), Relational Operator/1
  Delay1/1 -> Block RAM/3(wr_en), AND/1
  Delay2/1 -> Multiport Switch1/1
  Relational Operator/1 -> AND/2
  Vote/1 -> Add/1
  Zero/1 -> Multiport Switch/2

== system gm_parallel_lht/Parallel LHT/Parallel LHT Accumulator/Accumulator with Switches/Accumulator_instance98 ==
  mode : Inport  OutDataTypeStr=boolean  PortDimensions=1  SampleTime=6.66666666666667e-09
  address : Inport  Port=2  OutDataTypeStr=fixdt(0, 11, 0)  PortDimensions=1  SampleTime=6.66666666666667e-09
  edge : Inport  Port=3  OutDataTypeStr=boolean  PortDimensions=1  SampleTime=6.66666666666667e-09
  AND : Logic  IconShape=distinctive  AllPortsSameDT=off  OutDataTypeStr=boolean
  Add : Sum  OutDataTypeStr=fixdt(0, ceil(log2(maxRho*2)), 0)
  Block RAM : Subsystem
  Delay{,1..3} (4 alike) : Delay  DelayLength=1
  Multiport Switch : MultiPortSwitch  DataPortOrder=Zero-based contiguous  Inputs=2  zeroidx=on
  Multiport Switch1 : MultiPortSwitch  DataPortOrder=Zero-based contiguous  Inputs=2  zeroidx=on
  Relational Operator : RelationalOperator  Operator===  OutDataTypeStr=boolean  RndMeth=Simplest
  Vote : Constant  OutDataTypeStr=fixdt(0,1,0)  SampleTime=-1
  Zero : Constant  OutDataTypeStr=fixdt(0,1,0)  SampleTime=-1
  hps : Outport
  wires:
  Add/1 -> Delay3/1, Multiport Switch/3
  Multiport Switch1/1 -> Add/2
  Delay3/1 -> Multiport Switch1/3
  Multiport Switch/1 -> Block RAM/1(wr_data)
  edge/1 -> Delay1/1
  address/1 -> Block RAM/4(rd_addr), Delay/1, Relational Operator/2
  mode/1 -> Multiport Switch/1
  AND/1 -> Delay2/1
  Block RAM/1(rd_data) -> Multiport Switch1/2, hps/1
  Delay/1 -> Block RAM/2(wr_addr), Relational Operator/1
  Delay1/1 -> Block RAM/3(wr_en), AND/1
  Delay2/1 -> Multiport Switch1/1
  Relational Operator/1 -> AND/2
  Vote/1 -> Add/1
  Zero/1 -> Multiport Switch/2

== system gm_parallel_lht/Parallel LHT/Parallel LHT Accumulator/Accumulator with Switches/Accumulator_instance99 ==
  mode : Inport  OutDataTypeStr=boolean  PortDimensions=1  SampleTime=6.66666666666667e-09
  address : Inport  Port=2  OutDataTypeStr=fixdt(0, 11, 0)  PortDimensions=1  SampleTime=6.66666666666667e-09
  edge : Inport  Port=3  OutDataTypeStr=boolean  PortDimensions=1  SampleTime=6.66666666666667e-09
  AND : Logic  IconShape=distinctive  AllPortsSameDT=off  OutDataTypeStr=boolean
  Add : Sum  OutDataTypeStr=fixdt(0, ceil(log2(maxRho*2)), 0)
  Block RAM : Subsystem
  Delay{,1..3} (4 alike) : Delay  DelayLength=1
  Multiport Switch : MultiPortSwitch  DataPortOrder=Zero-based contiguous  Inputs=2  zeroidx=on
  Multiport Switch1 : MultiPortSwitch  DataPortOrder=Zero-based contiguous  Inputs=2  zeroidx=on
  Relational Operator : RelationalOperator  Operator===  OutDataTypeStr=boolean  RndMeth=Simplest
  Vote : Constant  OutDataTypeStr=fixdt(0,1,0)  SampleTime=-1
  Zero : Constant  OutDataTypeStr=fixdt(0,1,0)  SampleTime=-1
  hps : Outport
  wires:
  Add/1 -> Delay3/1, Multiport Switch/3
  Multiport Switch1/1 -> Add/2
  Delay3/1 -> Multiport Switch1/3
  Multiport Switch/1 -> Block RAM/1(wr_data)
  edge/1 -> Delay1/1
  address/1 -> Block RAM/4(rd_addr), Delay/1, Relational Operator/2
  mode/1 -> Multiport Switch/1
  AND/1 -> Delay2/1
  Block RAM/1(rd_data) -> Multiport Switch1/2, hps/1
  Delay/1 -> Block RAM/2(wr_addr), Relational Operator/1
  Delay1/1 -> Block RAM/3(wr_en), AND/1
  Delay2/1 -> Multiport Switch1/1
  Relational Operator/1 -> AND/2
  Vote/1 -> Add/1
  Zero/1 -> Multiport Switch/2

== system gm_parallel_lht/Parallel LHT/Parallel LHT Kernel/Hough Kernel/Hough Kernel Symmetric Look Ahead ==
  X : Inport  OutDataTypeStr=fixdt(1, 10, 0)  PortDimensions=1  SampleTime=6.66666666666667e-09
  Y : Inport  Port=2  OutDataTypeStr=fixdt(1, 10, 0)  PortDimensions=1  SampleTime=6.66666666666667e-09
  Compare To Constant1 : simulink/Logic and Bit Operations/Compare To Constant  relop===  const=width/2-1  OutDataTypeStr=boolean
  Hough Kernel Symmetric : Subsystem
  Look Ahead Hough : Subsystem
  Rho : Outport  VectorParamsAs1DForOutWhenUnconnected=off
  wires:
  Compare To Constant1/1 -> Look Ahead Hough/2(eol)
  Hough Kernel Symmetric/1(Rho) -> Rho/1
  Look Ahead Hough/1(ysin) -> Hough Kernel Symmetric/2(ysin)
  X/1 -> Compare To Constant1/1, Hough Kernel Symmetric/1(X)
  Y/1 -> Look Ahead Hough/1(Y)
